simulink model "Lab4_2_sol"  (R2015a)
settings: Solver=ode45  StartTime=0.0  StopTime=30000/491.52e6  RelTol=1e-3
PreLoadFcn:
  | Lab3_init
undefined symbols (not defined in the file): AXI4, Lite, periodScale, xlfda_numerator
libraries: xbsIndex_r4 x21
settings Model: CovSFcnEnable=off  Creator=danielm  LastModifiedBy=duncanm
settings DataIOCC: SignalLoggingSaveFormat=ModelDataLogs
settings DebuggingCC: SolverPrmCheckMsg=warning  MultiTaskDSMMsg=warning  MultiTaskCondExecSysMsg=none

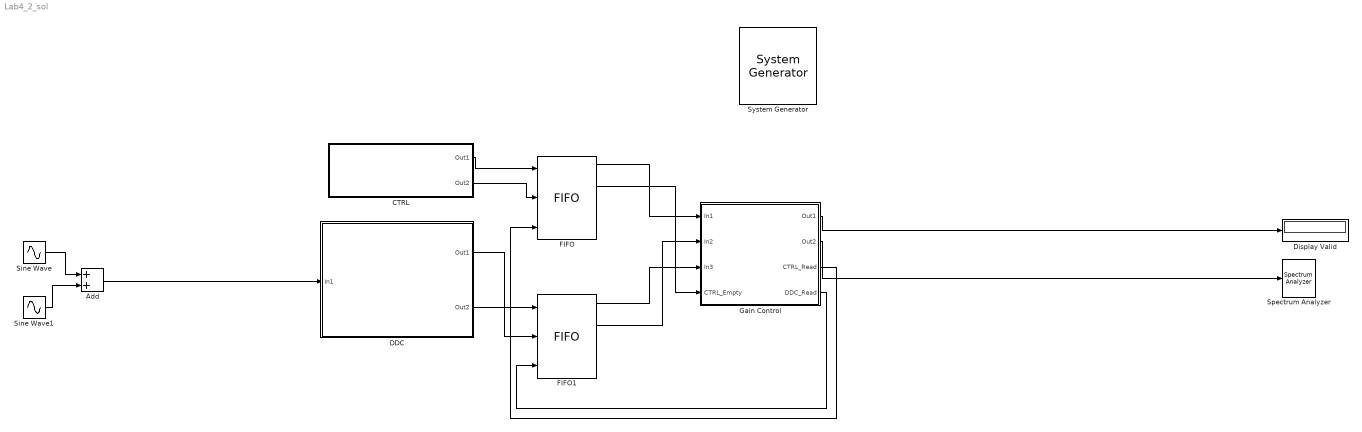
== system Lab4_2_sol ==
  " System Generator" : xbsIndex_r4/ System Generator  Tag=genX  xilinxfamily=zynq  part=xc7z045  speed=-2  package=ffg900  synthesis_tool=Vivado  clock_wrapper=Clock Enables  directory=./IPP_QT_MCD_0001/DDC_HB_hier  proj_type=Vivado  Synth_file=Vivado Synthesis Defaults  Impl_file=Vivado Implementation Defaults  testbench=on  simulink_period=1/491.52e6  sysclk_period=1e9/491.52e6  dcm_input_clock_period=10  incr_netlist=off  trim_vbits=Everywhere in SubSystem  dbl_ovrd=According to Block Masks  core_generation=According to Block Masks  run_coregen=off  deprecated_control=off  eval_field=0  block_type=sysgen
  Add : Sum
  "CTRL " : Subsystem
  DDC : Subsystem
  Display Valid : Display
  FIFO : xbsIndex_r4/FIFO  mem_type=Block RAM  performance_options=Standard_FIFO  embedded_registers=off  depth=16  percent_nbits=1  rst=off  rst_latency=1  en=off  use_dcount=off  use_percent_full_port=on  use_almost_empty=off  almost_empty_thresh=2  use_almost_full=off  almost_full_thresh=14  explicit_period=off  dbl_ovrd=off  block_type=fifo
  FIFO1 : xbsIndex_r4/FIFO  mem_type=Block RAM  performance_options=Standard_FIFO  embedded_registers=off  depth=16  percent_nbits=1  rst=off  rst_latency=1  en=off  use_dcount=off  use_percent_full_port=on  use_almost_empty=off  almost_empty_thresh=2  use_almost_full=off  almost_full_thresh=14  explicit_period=off  dbl_ovrd=off  block_type=fifo
  Gain Control : Subsystem
  Sine Wave : Sin  Frequency=2*pi*20e6/periodScale  SampleTime=0
  Sine Wave1 : Sin  Amplitude=0.25  Frequency=2*pi*1e6/periodScale  SampleTime=0
  Spectrum Analyzer : SpectrumAnalyzer
  wires:
  Sine Wave/1 -> Add/1
  Sine Wave1/1 -> Add/2
  Add/1 -> DDC/1(In1)
  Gain Control/1(Out1) -> Display Valid/1
  Gain Control/2(Out2) -> Spectrum Analyzer/1
  "CTRL "/1(Out1) -> FIFO/1
  FIFO/1 -> Gain Control/1(In1)
  DDC/2(Out2) -> FIFO1/1
  FIFO1/1 -> Gain Control/3(In3)
  "CTRL "/2(Out2) -> FIFO/2
  DDC/1(Out1) -> FIFO1/2
  FIFO/2 -> Gain Control/4(CTRL_Empty)
  Gain Control/3(CTRL_Read) -> FIFO/3
  Gain Control/4(DDC_Read) -> FIFO1/3
  FIFO1/2 -> Gain Control/2(In2)

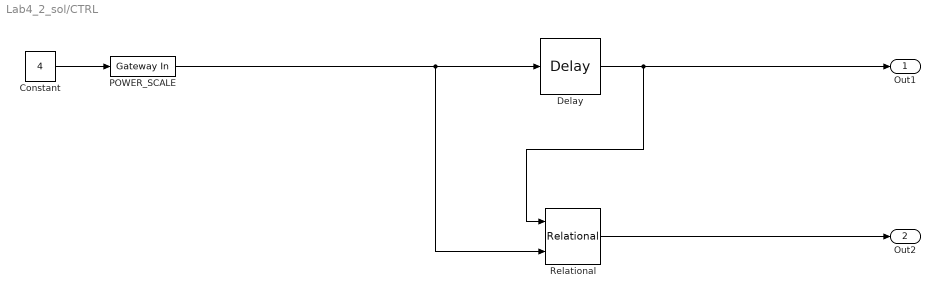
== system Lab4_2_sol/CTRL  ==
  Constant : Constant  Value=4
  Delay : xbsIndex_r4/Delay  rst=off  infoeditControl=Selection of Reset will increase slice count due to use of real FFs and instead of SRLs  en=off  latency=1  reg_retiming=off  dbl_ovrd=off  block_type=delay
  POWER_SCALE : xbsIndex_r4/Gateway In  gui_display_data_type=Fixed-point  arith_type=Unsigned  n_bits=inReg_0_NBits  bin_pt=inReg_0_BinPt  preci_type=Single  exp_width=8  frac_width=24  rows=1  columns=1  quantization="Round  (unbiased: +/- Inf)"  overflow=Saturate  period=8/491.52e6  UseAsADC=off  ADCChannel='1'  interface=AXI4-Lite  automatic_assignment=on  address_offset=hex2dec('00')  intf_name=''  intf_description=''  timing_constraint=None  locs_specified=off  LOCs={}  io_standard={}  inherit_from_input=off  hdl_port=on  dbl_ovrd=off  block_type=gatewayin
  Relational : xbsIndex_r4/Relational  mode=a!=b  op_type=Bool  en=off  latency=1  dbl_ovrd=off  block_type=relational
  Out1 : Outport
  Out2 : Outport  Port=2
  wires:
  Constant/1 -> POWER_SCALE/1
  POWER_SCALE/1 -> Relational/2, Delay/1
  Delay/1 -> Relational/1, Out1/1
  Relational/1 -> Out2/1

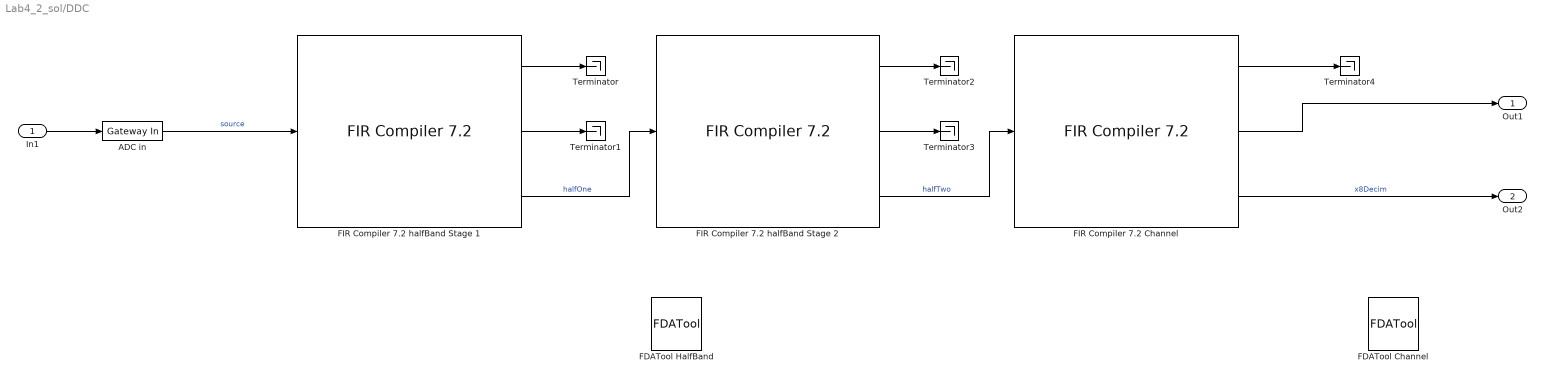
== system Lab4_2_sol/DDC ==
  In1 : Inport
  ADC in : xbsIndex_r4/Gateway In  gui_display_data_type=Fixed-point  arith_type="Signed  (2's comp)"  n_bits=16  bin_pt=14  preci_type=Single  exp_width=8  frac_width=24  rows=1  columns=1  quantization="Round  (unbiased: +/- Inf)"  overflow=Saturate  period=1/491.52e6  UseAsADC=off  ADCChannel='1'  interface=None  automatic_assignment=on  address_offset=hex2dec('00')  intf_name=''  intf_description=''  timing_constraint=None  locs_specified=off  LOCs={}  io_standard={}  inherit_from_input=off  hdl_port=on  dbl_ovrd=off  block_type=gatewayin
  FDATool Channel : xbsIndex_r4/FDATool  block_type=fdatool
      settings: infoedit=FDATool
  FDATool HalfBand : xbsIndex_r4/FDATool  block_type=fdatool
      settings: infoedit=FDATool
  FIR Compiler 7.2 Channel : xbsIndex_r4/FIR Compiler 7.2   coefficientvector=xlfda_numerator('FDATool Channel')  coefficient_sets=1  coefficient_reload=off  filter_type=Decimation  rate_change_type=Integer  interpolation_rate=1  decimation_rate=2  zero_pack_factor=1  channel_sequence=Basic  number_channels=1  pattern_list='P4-0,P4-1,P4-2,P4-3,P4-4'  number_paths=1  ratespecification=Maximum_Possible  sampleperiod=4  hardwareoversamplingrate=1  coefficient_sign=Signed  quantization=Quantize_Only  coefficient_width=16  bestprecision=on  coefficient_fractional_bits=18  coefficient_structure=Inferred  output_rounding_mode=Truncate_LSBs  output_width=22  filter_architecture=Systolic_Multiply_Accumulate  optimization_goal=Area  optimization_list='None'  data_buffer_type=Automatic  coefficient_buffer_type=Automatic  input_buffer_type=Automatic  output_buffer_type=Automatic  preference_for_other_storage=Automatic  multi_column_support=Automatic  columnconfig='32'  inter_column_pipe_length=4  data_has_tlast=Not_Required  m_data_has_tready=off  s_data_has_fifo=off  s_data_has_tuser=Not_Required  m_data_has_tuser=Not_Required  s_config_sync_mode=On_Vector  s_config_method=Single  num_reload_slots=1  has_aclken=off  has_aresetn=off  infoeditControl=ARESETn must be asserted for a minimum of 2 cycles  reset_data_vector=on  trim_axipin_name=on  simulation_type=hybrid_sim  simulation_model=sysgen:xfirv7_2_cmodel  data_path_portlist={ 's_axis_data_tdata', 'm_axis_data_tdata' }  passband_min=0.0  passband_max=0.5  stopband_min=0.5  stopband_max=1.0  filter_selection=1  gui_behaviour='Sysgen_GUI'  data_sign=Signed  data_width=16  data_fractional_bits=0  data_tuser_width=1  wrapper_available=true  ip_wrap_arbitrary_binary_point=true  ip_name=FIR Compiler  ip_version=7.2  dsptool_ready=true  ipcore_usecache=true  ipcore_useipmodelcache=true  port_translation_map={ 'aclken' => 'en', 'aresetn' => 'rst' }  run_core_at_system_period=true  ipcore_xco_need_fpga_part=true  block_type=fir_compiler_v7_2
      settings: infoedit=Maximum Possible : Maximizes oversampling rate. Abstracted input handshake (no s_data_tvalid) and automatic rate propagation.<br>Hardware Oversampling Rate : Specifies oversampling rate relative to the input sample period. Abstracted input handshake (no s_data_tvalid) and automatic rate propagation.<br>Input/Output Sample Period : Specifies absolute oversampling rate. No input handshake abstraction (exposes s_data_tvalid) and no rate propagation.
  FIR Compiler 7.2 halfBand Stage 2 : xbsIndex_r4/FIR Compiler 7.2   coefficientvector=xlfda_numerator('FDATool HalfBand')  coefficient_sets=1  coefficient_reload=off  filter_type=Decimation  rate_change_type=Integer  interpolation_rate=1  decimation_rate=2  zero_pack_factor=1  channel_sequence=Basic  number_channels=1  pattern_list='P4-0,P4-1,P4-2,P4-3,P4-4'  number_paths=1  ratespecification=Maximum_Possible  sampleperiod=2  hardwareoversamplingrate=1  coefficient_sign=Signed  quantization=Quantize_Only  coefficient_width=16  bestprecision=off  coefficient_fractional_bits=15  coefficient_structure=Inferred  output_rounding_mode=Non_Symmetric_Rounding_Down  output_width=22  filter_architecture=Systolic_Multiply_Accumulate  optimization_goal=Area  optimization_list='None'  data_buffer_type=Automatic  coefficient_buffer_type=Automatic  input_buffer_type=Automatic  output_buffer_type=Automatic  preference_for_other_storage=Automatic  multi_column_support=Automatic  columnconfig='1'  inter_column_pipe_length=4  data_has_tlast=Not_Required  m_data_has_tready=off  s_data_has_fifo=off  s_data_has_tuser=Not_Required  m_data_has_tuser=Not_Required  s_config_sync_mode=On_Vector  s_config_method=Single  num_reload_slots=1  has_aclken=off  has_aresetn=off  infoeditControl=ARESETn must be asserted for a minimum of 2 cycles  reset_data_vector=on  trim_axipin_name=on  simulation_type=hybrid_sim  simulation_model=sysgen:xfirv7_2_cmodel  data_path_portlist={ 's_axis_data_tdata', 'm_axis_data_tdata' }  passband_min=0.0  passband_max=0.5  stopband_min=0.5  stopband_max=1.0  filter_selection=1  gui_behaviour='Sysgen_GUI'  data_sign=Signed  data_width=16  data_fractional_bits=0  data_tuser_width=1  wrapper_available=true  ip_wrap_arbitrary_binary_point=true  ip_name=FIR Compiler  ip_version=7.2  dsptool_ready=true  ipcore_usecache=true  ipcore_useipmodelcache=true  port_translation_map={ 'aclken' => 'en', 'aresetn' => 'rst' }  run_core_at_system_period=true  ipcore_xco_need_fpga_part=true  block_type=fir_compiler_v7_2
      settings: infoedit=Maximum Possible : Maximizes oversampling rate. Abstracted input handshake (no s_data_tvalid) and automatic rate propagation.<br>Hardware Oversampling Rate : Specifies oversampling rate relative to the input sample period. Abstracted input handshake (no s_data_tvalid) and automatic rate propagation.<br>Input/Output Sample Period : Specifies absolute oversampling rate. No input handshake abstraction (exposes s_data_tvalid) and no rate propagation.
  FIR Compiler 7.2 halfBand Stage 1 : xbsIndex_r4/FIR Compiler 7.2   coefficientvector=xlfda_numerator('FDATool HalfBand')  coefficient_sets=1  coefficient_reload=off  filter_type=Decimation  rate_change_type=Integer  interpolation_rate=1  decimation_rate=2  zero_pack_factor=1  channel_sequence=Basic  number_channels=1  pattern_list='P4-0,P4-1,P4-2,P4-3,P4-4'  number_paths=1  ratespecification=Maximum_Possible  sampleperiod=2  hardwareoversamplingrate=1  coefficient_sign=Signed  quantization=Quantize_Only  coefficient_width=16  bestprecision=off  coefficient_fractional_bits=15  coefficient_structure=Inferred  output_rounding_mode=Non_Symmetric_Rounding_Down  output_width=22  filter_architecture=Systolic_Multiply_Accumulate  optimization_goal=Area  optimization_list='None'  data_buffer_type=Automatic  coefficient_buffer_type=Automatic  input_buffer_type=Automatic  output_buffer_type=Automatic  preference_for_other_storage=Automatic  multi_column_support=Automatic  columnconfig='1'  inter_column_pipe_length=4  data_has_tlast=Not_Required  m_data_has_tready=off  s_data_has_fifo=off  s_data_has_tuser=Not_Required  m_data_has_tuser=Not_Required  s_config_sync_mode=On_Vector  s_config_method=Single  num_reload_slots=1  has_aclken=off  has_aresetn=off  infoeditControl=ARESETn must be asserted for a minimum of 2 cycles  reset_data_vector=on  trim_axipin_name=on  simulation_type=hybrid_sim  simulation_model=sysgen:xfirv7_2_cmodel  data_path_portlist={ 's_axis_data_tdata', 'm_axis_data_tdata' }  passband_min=0.0  passband_max=0.5  stopband_min=0.5  stopband_max=1.0  filter_selection=1  gui_behaviour='Sysgen_GUI'  data_sign=Signed  data_width=16  data_fractional_bits=0  data_tuser_width=1  wrapper_available=true  ip_wrap_arbitrary_binary_point=true  ip_name=FIR Compiler  ip_version=7.2  dsptool_ready=true  ipcore_usecache=true  ipcore_useipmodelcache=true  port_translation_map={ 'aclken' => 'en', 'aresetn' => 'rst' }  run_core_at_system_period=true  ipcore_xco_need_fpga_part=true  block_type=fir_compiler_v7_2
      settings: infoedit=Maximum Possible : Maximizes oversampling rate. Abstracted input handshake (no s_data_tvalid) and automatic rate propagation.<br>Hardware Oversampling Rate : Specifies oversampling rate relative to the input sample period. Abstracted input handshake (no s_data_tvalid) and automatic rate propagation.<br>Input/Output Sample Period : Specifies absolute oversampling rate. No input handshake abstraction (exposes s_data_tvalid) and no rate propagation.
  Terminator{,1..4} (5 alike) : Terminator
  Out1 : Outport
  Out2 : Outport  Port=2
  wires:
  In1/1 -> ADC in/1
  ADC in/1 -> FIR Compiler 7.2 halfBand Stage 1/1  "source"
  FIR Compiler 7.2 halfBand Stage 1/3 -> FIR Compiler 7.2 halfBand Stage 2/1  "halfOne"
  FIR Compiler 7.2 halfBand Stage 2/3 -> FIR Compiler 7.2 Channel/1  "halfTwo"
  FIR Compiler 7.2 Channel/3 -> Out2/1  "x8Decim"
  FIR Compiler 7.2 halfBand Stage 2/1 -> Terminator2/1
  FIR Compiler 7.2 halfBand Stage 1/2 -> Terminator1/1
  FIR Compiler 7.2 halfBand Stage 2/2 -> Terminator3/1
  FIR Compiler 7.2 Channel/1 -> Terminator4/1
  FIR Compiler 7.2 halfBand Stage 1/1 -> Terminator/1
  FIR Compiler 7.2 Channel/2 -> Out1/1

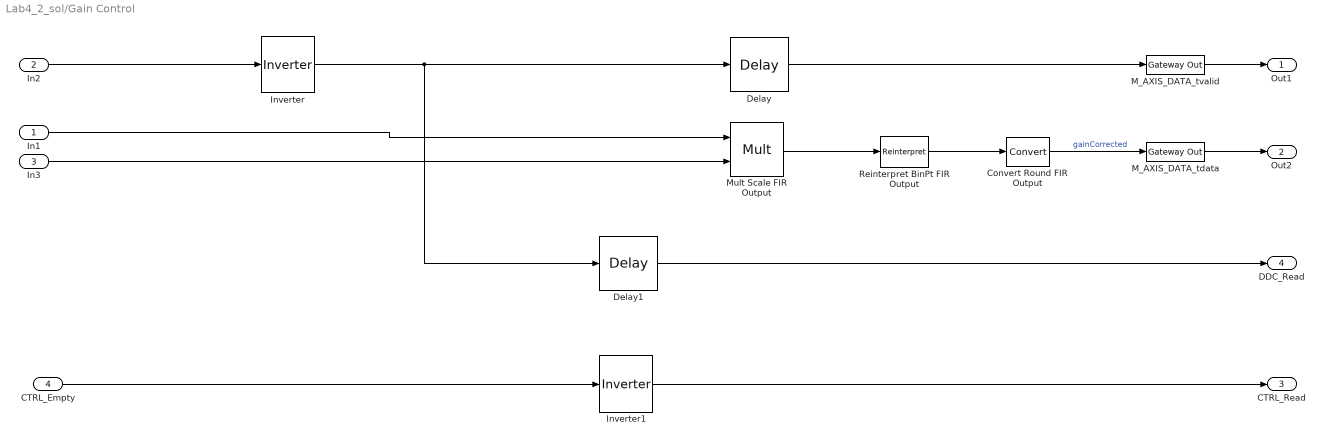
== system Lab4_2_sol/Gain Control ==
  In1 : Inport
  In2 : Inport  Port=2
  In3 : Inport  Port=3
  CTRL_Empty : Inport  Port=4
  Convert Round FIR Output : xbsIndex_r4/Convert  gui_display_data_type=Fixed-point  arith_type="Signed  (2's comp)"  n_bits=16  bin_pt=14  float_type=Single  exp_bits=8  fraction_bits=24  quantization="Round  (unbiased: +/- Inf)"  overflow=Saturate  en=off  latency=3  pipeline=off  dbl_ovrd=off  block_type=convert
  Delay : xbsIndex_r4/Delay  rst=off  infoeditControl=Selection of Reset will increase slice count due to use of real FFs and instead of SRLs  en=off  latency=6  reg_retiming=off  dbl_ovrd=off  block_type=delay
  Delay1 : xbsIndex_r4/Delay  rst=off  infoeditControl=Selection of Reset will increase slice count due to use of real FFs and instead of SRLs  en=off  latency=1  reg_retiming=off  dbl_ovrd=off  block_type=delay
  Inverter : xbsIndex_r4/Inverter  en=off  latency=1  dbl_ovrd=off  block_type=inv
  Inverter1 : xbsIndex_r4/Inverter  en=off  latency=1  dbl_ovrd=off  block_type=inv
  M_AXIS_DATA_tdata : xbsIndex_r4/Gateway Out  inherit_from_input=off  hdl_port=on  rows=1  columns=1  UseAsDAC=off  DACChannel='1'  interface=None  automatic_assignment=on  address_offset=hex2dec('00')  intf_name=''  intf_description=''  timing_constraint=None  locs_specified=off  LOCs={}  io_standard={}  block_type=gatewayout
  M_AXIS_DATA_tvalid : xbsIndex_r4/Gateway Out  inherit_from_input=off  hdl_port=on  rows=1  columns=1  UseAsDAC=off  DACChannel='1'  interface=None  automatic_assignment=on  address_offset=hex2dec('00')  intf_name=''  intf_description=''  timing_constraint=None  locs_specified=off  LOCs={}  io_standard={}  block_type=gatewayout
  Mult Scale FIR Output : xbsIndex_r4/Mult  precision=Full  arith_type="Signed  (2's comp)"  n_bits=16  bin_pt=14  quantization=Truncate  overflow=Saturate  en=off  latency=3  use_behavioral_HDL=off  opt=Speed  use_embedded=on  optimum_pipeline=off  pipeline=on  dbl_ovrd=off  use_rpm=on  placement_style=Triangular  block_type=mult
  Reinterpret BinPt FIR Output : xbsIndex_r4/Reinterpret  force_arith_type=off  arith_type=Unsigned  force_bin_pt=off  bin_pt=0  block_type=reinterpret
  Out1 : Outport
  Out2 : Outport  Port=2
  CTRL_Read : Outport  Port=3
  DDC_Read : Outport  Port=4
  wires:
  M_AXIS_DATA_tvalid/1 -> Out1/1
  M_AXIS_DATA_tdata/1 -> Out2/1
  Delay/1 -> M_AXIS_DATA_tvalid/1
  In1/1 -> Mult Scale FIR Output/1
  Mult Scale FIR Output/1 -> Reinterpret BinPt FIR Output/1
  Convert Round FIR Output/1 -> M_AXIS_DATA_tdata/1  "gainCorrected"
  Reinterpret BinPt FIR Output/1 -> Convert Round FIR Output/1
  In3/1 -> Mult Scale FIR Output/2
  In2/1 -> Inverter/1
  Inverter/1 -> Delay1/1, Delay/1
  Delay1/1 -> DDC_Read/1
  CTRL_Empty/1 -> Inverter1/1
  Inverter1/1 -> CTRL_Read/1
